simulink library "ProductionLineLib_CM"  (R2025a)
settings: Solver=VariableStepAuto  StartTime=0.0  StopTime=10.0  RelTol=1e-3
libraries: NSA_DEVS_MATH_OPERATIONS x72, $bdroot x37, NSA_DEVS_SOURCES x23, ProductionLineLib_AM x7, NSA_DEVS_DIGITALI3E_CONVERTER x6, NSA_DEVS_STATISTICS x5, NSA_DEVS_QSS x5, NSA_DEVS_ROUTING x4, NSA_DEVS_LOGISTICS x3
(part 1 of 2)
settings Model: Creator=peter  LastModifiedBy=peter
settings RTWCC: GPUComputeCapability=3.5

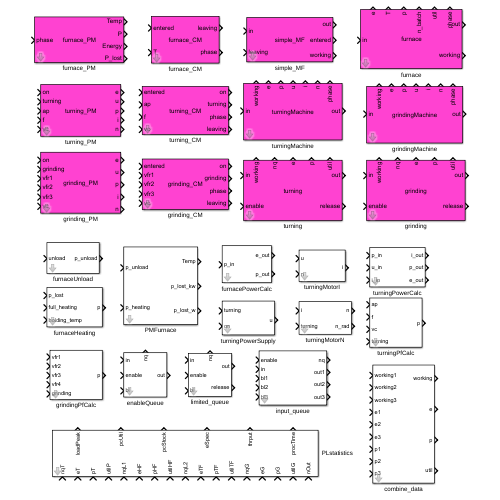
[thumbnail: Simulink's stored preview of the top-level diagram]
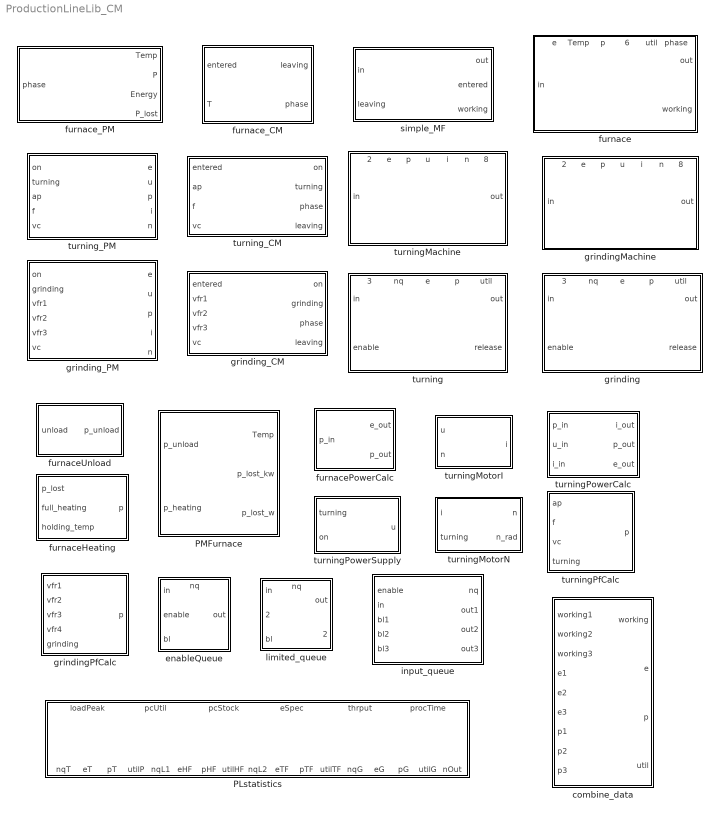
== system ProductionLineLib_CM ==
  PLstatistics : Subsystem  mask{tau=[0,1], debug=0}
      mask DialogControl Container2 Prompt: Advanced
  PMFurnace : Subsystem  mask{Te=0, Co=0, k_A=0, tauInt=[0,100], tau=[0,1], debug=0}
      mask prompts: tauInt "input delay of integrators"
      mask DialogControl Container3 Prompt: General
      mask DialogControl Container2 Prompt: Advanced
  combine_data : Subsystem  mask{tau=[0,1], debug=0}
      mask DialogControl Container3 Prompt: Advanced
  enableQueue : Subsystem  mask{tD=[0,2], tau=[0,1], debug=0}
      mask prompts: tD "delay time of the queuingFree state"
      settings: PortSchema="{\"entries\":[{\"content\":{\"sides\":[{\"content\":{\"connectorIds\":[\"In1\",\"In2\",\"In3\"]},\"type\":\"ConnectorPlacement.EquallySpacedRectSide\",\"uuid\":\"2ad8f87e-7312-4304-b0af-e4f2759959c2\"},{\"content\":{\"connectorIds\":[\"Out1\"],\"side\":\"RIGHT\"},\"type\":\"ConnectorPlacement.EquallySpacedRectSide\",\"uuid\":\"09964865-65de-4b09-b55b-65dbc64d6c80\"},{\"content\":{\"connectorIds\":[\"Out2\"],\"side\":\"TOP\"},\"type\":\"ConnectorPlacement.EquallySpacedRectSide\",\"uuid\":\"570c44b6-46bf-4374-8bed-d6fd4de2ba36\"}]},\"type\":\"ConnectorPlacement.EquallySpacedConnector\",\"uuid\":\"08fead9e-e551-4d6e-a21e-4bd06ec318c1\"}],\"packageUris\":[\"http://schema.mathworks.com/mf0/Connector/R2020b\"],\"version\":\"1.0\"}"
      mask DialogControl Container4 Prompt: Advanced
  furnace : Subsystem  mask{PH=0, Co=0, k_A=0, Te=0, P0=0, P_unload=0, holding_time=0, Tsoll=0, Kapa=0, tauInt=[0,100], tauCont=[0,100], tau=[0,1], debug=0}
      mask prompts: tauInt "input delay of integrators"; tauCont "input delay of controllers"
      settings: PortSchema="{\"entries\":[{\"content\":{\"sides\":[{\"content\":{\"connectorIds\":[\"In1\"]},\"type\":\"ConnectorPlacement.EquallySpacedRectSide\",\"uuid\":\"48eb3c0c-68de-4a57-9b4e-df051f691ee9\"},{\"content\":{\"connectorIds\":[\"Out1\",\"Out2\"],\"side\":\"RIGHT\"},\"type\":\"ConnectorPlacement.EquallySpacedRectSide\",\"uuid\":\"00e094f9-0571-45d6-b681-fd41a6529743\"},{\"content\":{\"connectorIds\":[\"Out3\",\"Out4\",\"Out5\",\"Out6\",\"Out7\",\"Out8\"],\"side\":\"TOP\"},\"type\":\"ConnectorPlacement.EquallySpacedRectSide\",\"uuid\":\"550a95d5-71f4-45dc-b750-a4b185df31ac\"}]},\"type\":\"ConnectorPlacement.EquallySpacedConnector\",\"uuid\":\"8d29a545-a928-42f4-bfc0-37c916a5d15f\"}],\"packageUris\":[\"http://schema.mathworks.com/mf0/Connector/R2020b\"],\"version\":\"1.0\"}"
      mask DialogControl Container2 Prompt: General
      mask DialogControl Container3 Prompt: Advanced
      mask Display:
      | disp('furnace');
      | port_label('input', 1, 'in');
      | 
      | port_label('output', 1, 'out');
      | port_label('output', 2, 'working');
      | port_label('output', 3, 'e');
      | port_label('output', 4, 'T');
      | port_label('output', 5, 'p');
      | port_label('output', 6, 'n_batch');
      | port_label('output', 7, 'util');
      | port_label('output', 8, 'phase');
  furnaceHeating : Subsystem  mask{tau=[0,1], debug=0, PH=0}
      mask DialogControl Container3 Prompt: General
      mask DialogControl Container2 Prompt: Advanced
  furnacePowerCalc : Subsystem  mask{P0=0, tauInt=[0,100], tau=[0,1], debug=0}
      mask prompts: tauInt "input delay of integrators"
      mask DialogControl Container3 Prompt: General
      mask DialogControl Container2 Prompt: Advanced
  furnaceUnload : Subsystem  mask{P_unload=0, tau=[0,1], debug=0}
      mask DialogControl Container3 Prompt: General
      mask DialogControl Container2 Prompt: Advanced
  furnace_CM : Subsystem  mask{holding_time=0, Tsoll=0, tau=[0,1], debug=0}
      mask DialogControl Container2 Prompt: General
      mask DialogControl Container3 Prompt: Advanced
      mask Display:
      | disp('furnace_CM');
      | port_label('input', 1, 'entered');
      | port_label('input', 2, 'T');
      | 
      | port_label('output', 1, 'leaving');
      | port_label('output', 2, 'phase');
  furnace_PM : Subsystem  mask(Furnace_PM){Te=0, P0=0, Co=0, PH=0, k_A=0, P_unload=0, tauInt=[0,100], tauCont=[0,100], tau=[0,1], debug=0}
      mask prompts: tauInt "input delay of integrators"; tauCont "input delay of controllers"
      mask help: Process model of a furnace.
      mask DialogControl Container3 Prompt: General
      mask DialogControl Container2 Prompt: Advanced
      mask Display:
      | disp('furnace_PM');
      | port_label('input', 1, 'phase');
      | 
      | port_label('output', 1, 'Temp');
      | port_label('output', 2, 'P');
      | port_label('output', 3, 'Energy');
      | port_label('output', 4, 'P_lost');
  grinding : Subsystem  mask{vfr1=0.5, vfr2=0.2, vfr3=0.03, vc=10, max_fifo=200, grinding_time=100, tauInt=[0,100], tauCont=[0,100], tau=[0,1], debug=0}
      mask prompts: grinding_time "grinding time"; tauInt "input delay of integrators"; tauCont "input delay of controllers"
      settings: PortSchema="{\"entries\":[{\"content\":{\"sides\":[{\"content\":{\"connectorIds\":[\"In1\",\"In2\"]},\"type\":\"ConnectorPlacement.EquallySpacedRectSide\",\"uuid\":\"33cbe9ec-8ffd-4808-aa33-03a03d7697b3\"},{\"content\":{\"connectorIds\":[\"Out1\",\"Out2\"],\"side\":\"RIGHT\"},\"type\":\"ConnectorPlacement.EquallySpacedRectSide\",\"uuid\":\"c4625700-92c7-457c-b718-8001350e1d76\"},{\"content\":{\"connectorIds\":[\"Out3\",\"Out4\",\"Out5\",\"Out6\",\"Out7\"],\"side\":\"TOP\"},\"type\":\"ConnectorPlacement.EquallySpacedRectSide\",\"uuid\":\"e2440e2f-ad0a-4c1e-a3bb-510435ac270c\"}]},\"type\":\"ConnectorPlacement.EquallySpacedConnector\",\"uuid\":\"8074284e-cd52-45ef-a5c6-c1af8e64b890\"}],\"packageUris\":[\"http://schema.mathworks.com/mf0/Connector/R2020b\"],\"version\":\"1.0\"}"
      mask DialogControl Container2 Prompt: General
      mask DialogControl Container3 Prompt: Advanced
      mask Display:
      | disp('grinding');
      | port_label('input', 1, 'in');
      | port_label('input', 2, 'enable');
      | 
      | port_label('output', 1, 'out');
      | port_label('output', 2, 'release');
      | port_label('output', 3, 'working');
      | port_label('output', 4, 'nq');
      | port_label('output', 5, 'e');
      | port_label('output', 6, 'p');
      | port_label('output', 7, 'util');
  grindingMachine : Subsystem  mask{grinding_time=0, vfr1_ug=0, vfr2_ug=0, vfr3_ug=0, vc_ug=0, vfr1_og=0, vfr2_og=0, vfr3_og=0, vc_og=0, P_vfr1=0, P_vfr2=0, P_vfr3=0, P_vc=0, vfr1=0, vfr2=0, vfr3=0, vc=0, tauInt=[0,100], tauCont=[0,100], tau=[0,1], debug=0}
      mask prompts: tauInt "input delay of integrators"; tauCont "input delay of controllers"
      settings: PortSchema="{\"entries\":[{\"content\":{\"sides\":[{\"content\":{\"connectorIds\":[\"In1\"]},\"type\":\"ConnectorPlacement.EquallySpacedRectSide\",\"uuid\":\"7ed7b3b0-123a-476c-9c35-5e38dde7b955\"},{\"content\":{\"connectorIds\":[\"Out1\"],\"side\":\"RIGHT\"},\"type\":\"ConnectorPlacement.EquallySpacedRectSide\",\"uuid\":\"8397d86f-174e-49cd-8a33-9d60b1d471dc\"},{\"content\":{\"connectorIds\":[\"Out2\",\"Out3\",\"Out4\",\"Out5\",\"Out6\",\"Out7\",\"Out8\"],\"side\":\"TOP\"},\"type\":\"ConnectorPlacement.EquallySpacedRectSide\",\"uuid\":\"d0d4c44f-158b-4425-aa76-17b6d066cd1d\"}]},\"type\":\"ConnectorPlacement.EquallySpacedConnector\",\"uuid\":\"e658c338-98e5-4f30-9f17-73625d396bbf\"}],\"packageUris\":[\"http://schema.mathworks.com/mf0/Connector/R2020b\"],\"version\":\"1.0\"}"
      mask DialogControl Container2 Prompt: General
      mask DialogControl Container3 Prompt: Advanced
      mask Display:
      | disp('grindingMachine');
      | port_label('input', 1, 'in');
      | 
      | port_label('output', 1, 'out');
      | port_label('output', 2, 'working');
      | port_label('output', 3, 'e');
      | port_label('output', 4, 'p');
      | port_label('output', 5, 'u');
      | port_label('output', 6, 'i');
      | port_label('output', 7, 'n');
      | port_label('output', 8, 'phase');
  grindingPfCalc : Subsystem  mask{vfr1_ug=0, vfr1_og=0, P_vfr1=0, vfr2_ug=0, vfr2_og=0, P_vfr2=0, vfr3_ug=0, vfr3_og=0, P_vfr3=0, vc_ug=0, vc_og=0, P_vc=0, tau=[0,1], debug=0}
      mask DialogControl Container3 Prompt: General
      mask DialogControl Container2 Prompt: Advanced
  grinding_CM : Subsystem  mask{grinding_time=0, vfr1_ug=0, vfr2_ug=0, vfr3_ug=0, vc_ug=0, vfr1_og=0, vfr2_og=0, vfr3_og=0, vc_og=0, tau=[0,100], debug=0}
      mask DialogControl Container2 Prompt: General
      mask DialogControl Container3 Prompt: Advanced
      mask Display:
      | disp('grinding_CM');
      | port_label('input', 1, 'entered');
      | port_label('input', 2, 'vfr1');
      | port_label('input', 3, 'vfr2');
      | port_label('input', 4, 'vfr3');
      | port_label('input', 5, 'vc');
      | 
      | port_label('output', 1, 'on');
      | port_label('output', 2, 'grinding');
      | port_label('output', 3, 'phase');
      | port_label('output', 4, 'leaving');
  grinding_PM : Subsystem  mask{R=0, L=0, J=0, b=0, K=0, vcc=0, vcc_load=0, load=0, vfr1_ug=0, vfr2_ug=0, vfr3_ug=0, vc_ug=0, vfr1_og=0, vfr2_og=0, vfr3_og=0, vc_og=0, P_vfr1=0, P_vfr2=0, P_vfr3=0, P_vc=0, tauInt=[0,100], tau=[0,1], debug=0}
      mask prompts: tauInt "input delay of integrators"
      mask DialogControl Container2 Prompt: General
      mask DialogControl Container3 Prompt: Advanced
      mask Display:
      | disp('grinding_PM');
      | port_label('input', 1, 'on');
      | port_label('input', 2, 'grinding');
      | port_label('input', 3, 'vfr1');
      | port_label('input', 4, 'vfr2');
      | port_label('input', 5, 'vfr3');
      | port_label('input', 6, 'vc');
      | 
      | port_label('output', 1, 'e');
      | port_label('output', 2, 'u');
      | port_label('output', 3, 'p');
      | port_label('output', 4, 'i');
      | port_label('output', 5, 'n');
  input_queue : Subsystem  mask{tD=[0,5], tau=[0,5], debug=0}
      mask prompts: tD "delay time of the queuingFree state"
      mask DialogControl Container3 Prompt: Advanced
  limited_queue : Subsystem  mask{max_fifo=400, tD=[0,5], tau=[0,5], debug=0}
      mask prompts: tD "delay time of the queuingFree state"
      settings: PortSchema="{\"entries\":[{\"content\":{\"sides\":[{\"content\":{\"connectorIds\":[\"In1\",\"In2\",\"In3\"]},\"type\":\"ConnectorPlacement.EquallySpacedRectSide\",\"uuid\":\"9e9b3e08-535a-451f-ab10-868cecb889f8\"},{\"content\":{\"connectorIds\":[\"Out1\",\"Out2\"],\"side\":\"RIGHT\"},\"type\":\"ConnectorPlacement.EquallySpacedRectSide\",\"uuid\":\"54afad95-e8b1-4ff2-82f7-3599ee077844\"},{\"content\":{\"connectorIds\":[\"Out3\"],\"side\":\"TOP\"},\"type\":\"ConnectorPlacement.EquallySpacedRectSide\",\"uuid\":\"41a9a62c-ac83-449a-b909-405f9dccd004\"}]},\"type\":\"ConnectorPlacement.EquallySpacedConnector\",\"uuid\":\"98ebd8e6-c994-4b03-9827-f562c62733d8\"}],\"packageUris\":[\"http://schema.mathworks.com/mf0/Connector/R2020b\"],\"version\":\"1.0\"}"
      mask DialogControl Container3 Prompt: General
      mask DialogControl Container2 Prompt: Advanced
  simple_MF : Subsystem  mask{tau=[0,1], debug=0}
      mask DialogControl Container2 Prompt: Advanced
      mask Display:
      | disp('simple_MF');
      | port_label('input', 1, 'in');
      | port_label('input', 2, 'leaving');
      | 
      | port_label('output', 1, 'out');
      | port_label('output', 2, 'entered');
      | port_label('output', 3, 'working');
  turning : Subsystem  mask{ap=1, f=0.1, vc=100, max_fifo=200, turning_time=100, tauInt=[0,100], tauCont=[0,100], tau=[0,1], debug=0}
      mask prompts: turning_time "turning time"; tauInt "input delay of integrators"; tauCont "input delay of controllers"
      settings: PortSchema="{\"entries\":[{\"content\":{\"sides\":[{\"content\":{\"connectorIds\":[\"In1\",\"In2\"]},\"type\":\"ConnectorPlacement.EquallySpacedRectSide\",\"uuid\":\"33cbe9ec-8ffd-4808-aa33-03a03d7697b3\"},{\"content\":{\"connectorIds\":[\"Out1\",\"Out2\"],\"side\":\"RIGHT\"},\"type\":\"ConnectorPlacement.EquallySpacedRectSide\",\"uuid\":\"c4625700-92c7-457c-b718-8001350e1d76\"},{\"content\":{\"connectorIds\":[\"Out3\",\"Out4\",\"Out5\",\"Out6\",\"Out7\"],\"side\":\"TOP\"},\"type\":\"ConnectorPlacement.EquallySpacedRectSide\",\"uuid\":\"e2440e2f-ad0a-4c1e-a3bb-510435ac270c\"}]},\"type\":\"ConnectorPlacement.EquallySpacedConnector\",\"uuid\":\"8074284e-cd52-45ef-a5c6-c1af8e64b890\"}],\"packageUris\":[\"http://schema.mathworks.com/mf0/Connector/R2020b\"],\"version\":\"1.0\"}"
      mask DialogControl Container2 Prompt: General
      mask DialogControl Container3 Prompt: Advanced
      mask Display:
      | disp('turning');
      | port_label('input', 1, 'in');
      | port_label('input', 2, 'enable');
      | 
      | port_label('output', 1, 'out');
      | port_label('output', 2, 'release');
      | port_label('output', 3, 'working');
      | port_label('output', 4, 'nq');
      | port_label('output', 5, 'e');
      | port_label('output', 6, 'p');
      | port_label('output', 7, 'util');
  turningMachine : Subsystem  mask{turning_time=0, ap_ug=0, ap_og=0, P_ap=0, f_ug=0, f_og=0, P_f=0, vc_ug=0, vc_og=0, P_vc=0, ap=0, f=0, vc=0, tauInt=[0,100], tauCont=[0,100], tau=[0,1], debug=0}
      mask prompts: tauInt "input delay of integrators"; tauCont "input delay of controllers"
      settings: PortSchema="{\"entries\":[{\"content\":{\"sides\":[{\"content\":{\"connectorIds\":[\"In1\"]},\"type\":\"ConnectorPlacement.EquallySpacedRectSide\",\"uuid\":\"7ed7b3b0-123a-476c-9c35-5e38dde7b955\"},{\"content\":{\"connectorIds\":[\"Out1\"],\"side\":\"RIGHT\"},\"type\":\"ConnectorPlacement.EquallySpacedRectSide\",\"uuid\":\"8397d86f-174e-49cd-8a33-9d60b1d471dc\"},{\"content\":{\"connectorIds\":[\"Out2\",\"Out3\",\"Out4\",\"Out5\",\"Out6\",\"Out7\",\"Out8\"],\"side\":\"TOP\"},\"type\":\"ConnectorPlacement.EquallySpacedRectSide\",\"uuid\":\"d0d4c44f-158b-4425-aa76-17b6d066cd1d\"}]},\"type\":\"ConnectorPlacement.EquallySpacedConnector\",\"uuid\":\"e658c338-98e5-4f30-9f17-73625d396bbf\"}],\"packageUris\":[\"http://schema.mathworks.com/mf0/Connector/R2020b\"],\"version\":\"1.0\"}"
      mask DialogControl Container2 Prompt: General
      mask DialogControl Container3 Prompt: Advanced
      mask Display:
      | disp('turningMachine');
      | port_label('input', 1, 'in');
      | 
      | port_label('output', 1, 'out');
      | port_label('output', 2, 'working');
      | port_label('output', 3, 'e');
      | port_label('output', 4, 'p');
      | port_label('output', 5, 'u');
      | port_label('output', 6, 'i');
      | port_label('output', 7, 'n');
      | port_label('output', 8, 'phase');
  turningMotorI : Subsystem  mask{R=0, L=0, K=0, tauInt=[0,100], tau=[0,1], debug=0}
      mask prompts: tauInt "input delay of integrators"
      mask DialogControl Container2 Prompt: General
      mask DialogControl Container3 Prompt: Advanced
  turningMotorN : Subsystem  mask{J=0, b=0, K=0, load=0, tauInt=[0,100], tau=[0,1], debug=0}
      mask prompts: tauInt "input delay of integrators"
      mask DialogControl Container2 Prompt: General
      mask DialogControl Container3 Prompt: Advanced
  turningPfCalc : Subsystem  mask{ap_ug=0, ap_og=0, P_ap=0, f_ug=0, f_og=0, P_f=0, vc_ug=0, vc_og=0, P_vc=0, tau=[0,1], debug=0}
      mask DialogControl Container3 Prompt: General
      mask DialogControl Container2 Prompt: Advanced
  turningPowerCalc : Subsystem  mask{tauInt=[0,100], tau=[0,1], debug=0}
      mask prompts: tauInt "input delay of integrators"
      mask DialogControl Container2 Prompt: Advanced
  turningPowerSupply : Subsystem  mask{vcc=0, vcc_load=0, tau=[0,1], debug=0}
      mask DialogControl Container2 Prompt: General
      mask DialogControl Container3 Prompt: Advanced
  turning_CM : Subsystem  mask{turning_time=0, ap_ug=0, f_ug=0, vc_ug=0, ap_og=0, f_og=0, vc_og=0, tau=[0,100], debug=0}
      mask DialogControl Container2 Prompt: General
      mask DialogControl Container3 Prompt: Advanced
      mask Display:
      | disp('turning_CM');
      | port_label('input', 1, 'entered');
      | port_label('input', 2, 'ap');
      | port_label('input', 3, 'f');
      | port_label('input', 4, 'vc');
      | 
      | port_label('output', 1, 'on');
      | port_label('output', 2, 'turning');
      | port_label('output', 3, 'phase');
      | port_label('output', 4, 'leaving');
  turning_PM : Subsystem  mask{R=0, L=0, J=0, b=0, K=0, vcc=0, vcc_load=0, load=0, ap_ug=0, f_ug=0, vc_ug=0, ap_og=0, f_og=0, vc_og=0, P_ap=0, P_f=0, P_vc=0, tauInt=[0,100], tau=[0,1], debug=0}
      mask prompts: tauInt "input delay of integrators"
      mask DialogControl Container2 Prompt: General
      mask DialogControl Container3 Prompt: Advanced
      mask Display:
      | disp('turning_PM');
      | port_label('input', 1, 'on');
      | port_label('input', 2, 'turning');
      | port_label('input', 3, 'ap');
      | port_label('input', 4, 'f');
      | port_label('input', 5, 'vc');
      | 
      | port_label('output', 1, 'e');
      | port_label('output', 2, 'u');
      | port_label('output', 3, 'p');
      | port_label('output', 4, 'i');
      | port_label('output', 5, 'n');

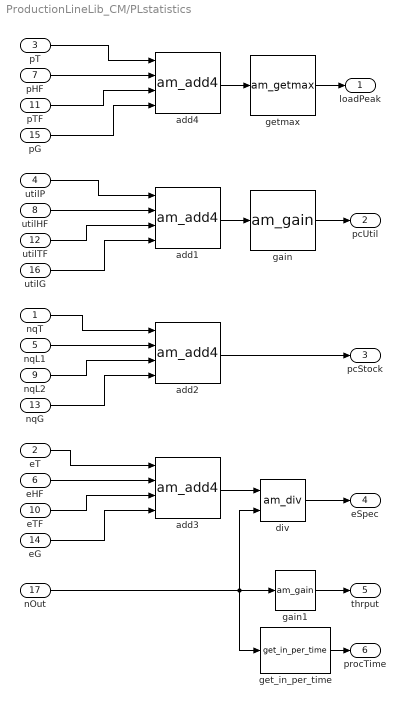
== system ProductionLineLib_CM/PLstatistics ==
  nqT : Inport
  eT : Inport  Port=2
  pT : Inport  Port=3
  utilP : Inport  Port=4
  nqL1 : Inport  Port=5
  eHF : Inport  Port=6
  pHF : Inport  Port=7
  utilHF : Inport  Port=8
  nqL2 : Inport  Port=9
  eTF : Inport  Port=10
  pTF : Inport  Port=11
  utilTF : Inport  Port=12
  nqG : Inport  Port=13
  eG : Inport  Port=14
  pG : Inport  Port=15
  utilG : Inport  Port=16
  nOut : Inport  Port=17
  add{1..4} (4 alike) : NSA_DEVS_MATH_OPERATIONS/am_add4  tau=[0,1]  debug=0
      settings: SourceProductName=Math Operations
  div : NSA_DEVS_MATH_OPERATIONS/am_div  tau=[0,1]  debug=0
      settings: SourceProductName=Math Operations
  gain : NSA_DEVS_MATH_OPERATIONS/am_gain  g=0.25  tau=[0,1]  debug=0
      settings: SourceProductName=Math Operations
  gain1 : NSA_DEVS_MATH_OPERATIONS/am_gain  g=1  tau=[0,1]  debug=0
      settings: SourceProductName=Math Operations
  get_in_per_time : ProductionLineLib_AM/get_in_per_time  tau=[0,1]  debug=0
  getmax : NSA_DEVS_STATISTICS/am_getmax  tau=[0,1]  debug=0
      settings: SourceProductName=Statistics
  loadPeak : Outport
  pcUtil : Outport  Port=2
  pcStock : Outport  Port=3
  eSpec : Outport  Port=4
  thrput : Outport  Port=5
  procTime : Outport  Port=6
  wires:
  pHF/1 -> add4/2
  nqL1/1 -> add2/2
  gain/1 -> pcUtil/1
  utilHF/1 -> add1/2
  add4/1 -> getmax/1
  eG/1 -> add3/4
  nOut/1 -> gain1/1, get_in_per_time/1, div/2
  utilTF/1 -> add1/3
  utilP/1 -> add1/1
  eHF/1 -> add3/2
  eT/1 -> add3/1
  add2/1 -> pcStock/1
  add1/1 -> gain/1
  pTF/1 -> add4/3
  nqT/1 -> add2/1
  nqL2/1 -> add2/3
  eTF/1 -> add3/3
  pG/1 -> add4/4
  pT/1 -> add4/1
  nqG/1 -> add2/4
  utilG/1 -> add1/4
  div/1 -> eSpec/1
  getmax/1 -> loadPeak/1
  add3/1 -> div/1
  get_in_per_time/1 -> procTime/1
  gain1/1 -> thrput/1

== system ProductionLineLib_CM/PMFurnace ==
  p_unload : Inport
  p_heating : Inport  Port=2
  add3 : NSA_DEVS_MATH_OPERATIONS/am_add3  tau=tau  debug=debug
      settings: SourceProductName=Math Operations
  am_add2 : NSA_DEVS_MATH_OPERATIONS/am_add2  tau=[0,1]  debug=0
      settings: SourceProductName=Math Operations
  am_const : NSA_DEVS_SOURCES/am_const  value=-Te  sendTime=[0,1]  debug=0
      settings: SourceProductName=Sources
  gain : NSA_DEVS_MATH_OPERATIONS/am_gain  g=1/Co  tau=[0,1]  debug=debug
      settings: SourceProductName=Math Operations
  gain1 : NSA_DEVS_MATH_OPERATIONS/am_gain  g=k_A  tau=[0,1]  debug=debug
      settings: SourceProductName=Math Operations
  gain2 : NSA_DEVS_MATH_OPERATIONS/am_gain  g=1/1000  tau=[0,1]  debug=debug
      settings: SourceProductName=Math Operations
  gain3 : NSA_DEVS_MATH_OPERATIONS/am_gain  g=-1  tau=[0,1]  debug=debug
      settings: SourceProductName=Math Operations
  hIntegrator : NSA_DEVS_QSS/am_hIntegrator  dq=25  epsilon=25  X0=Te  tau=tauInt  debug=debug
      settings: SourceProductName=QSS
  Temp : Outport
  p_lost_kw : Outport  Port=2
  p_lost_w : Outport  Port=3
  wires:
  hIntegrator/1 -> am_add2/2, Temp/1
  p_heating/1 -> add3/2
  p_unload/1 -> add3/1
  gain3/1 -> add3/3
  gain2/1 -> p_lost_kw/1
  am_add2/1 -> gain1/1
  gain1/1 -> gain2/1, p_lost_w/1, gain3/1
  am_const/1 -> am_add2/1
  gain/1 -> hIntegrator/1
  add3/1 -> gain/1

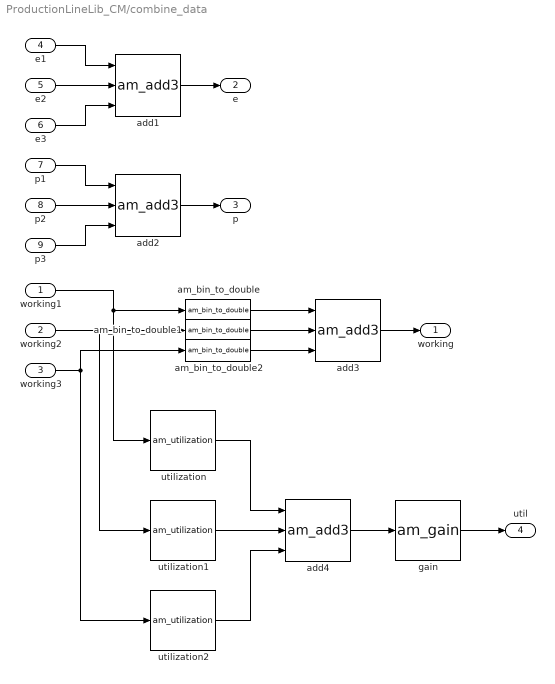
== system ProductionLineLib_CM/combine_data ==
  working1 : Inport
  working2 : Inport  Port=2
  working3 : Inport  Port=3
  e1 : Inport  Port=4
  e2 : Inport  Port=5
  e3 : Inport  Port=6
  p1 : Inport  Port=7
  p2 : Inport  Port=8
  p3 : Inport  Port=9
  add{1..4} (4 alike) : NSA_DEVS_MATH_OPERATIONS/am_add3  tau=[0,1]  debug=0
      settings: SourceProductName=Math Operations
  am_bin_to_double : NSA_DEVS_DIGITALI3E_CONVERTER/am_bin_to_double  tau=[0,1]  debug=0
  am_bin_to_double1 : NSA_DEVS_DIGITALI3E_CONVERTER/am_bin_to_double  tau=[0,1]  debug=0
  am_bin_to_double2 : NSA_DEVS_DIGITALI3E_CONVERTER/am_bin_to_double  tau=[0,1]  debug=0
  gain : NSA_DEVS_MATH_OPERATIONS/am_gain  g=1/3  tau=[0,1]  debug=0
      settings: SourceProductName=Math Operations
  utilization : NSA_DEVS_STATISTICS/am_utilization  tau=[0,1]  debug=0
      settings: SourceProductName=Statistics
  utilization1 : NSA_DEVS_STATISTICS/am_utilization  tau=[0,1]  debug=0
      settings: SourceProductName=Statistics
  utilization2 : NSA_DEVS_STATISTICS/am_utilization  tau=[0,1]  debug=0
      settings: SourceProductName=Statistics
  working : Outport
  e : Outport  Port=2
  p : Outport  Port=3
  util : Outport  Port=4
  wires:
  working2/1 -> utilization1/1, am_bin_to_double1/1
  working1/1 -> am_bin_to_double/1, utilization/1
  working3/1 -> am_bin_to_double2/1, utilization2/1
  add3/1 -> working/1
  e2/1 -> add1/2
  add1/1 -> e/1
  e1/1 -> add1/1
  e3/1 -> add1/3
  p2/1 -> add2/2
  p1/1 -> add2/1
  p3/1 -> add2/3
  add2/1 -> p/1
  utilization1/1 -> add4/2
  utilization/1 -> add4/1
  utilization2/1 -> add4/3
  add4/1 -> gain/1
  gain/1 -> util/1
  am_bin_to_double/1 -> add3/1
  am_bin_to_double1/1 -> add3/2
  am_bin_to_double2/1 -> add3/3

== system ProductionLineLib_CM/enableQueue ==
  in : Inport
  enable : Inport  Port=2
  bl : Inport  Port=3
  am_not1 : NSA_DEVS_MATH_OPERATIONS/am_not  i0=true  tau_copy=[0,1]  debug_copy=0
      settings: SourceProductName=Math Operations
  am_or2 : NSA_DEVS_MATH_OPERATIONS/am_or2  i0=false  tau_copy=[0,1]  debug_copy=0
      settings: SourceProductName=Math Operations
  queue : NSA_DEVS_LOGISTICS/am_queue  tD=tD  tau=tau  debug=debug
      settings: SourceProductName=Logistics
  out : Outport
  nq : Outport  Port=2
  wires:
  enable/1 -> am_not1/1
  am_not1/1 -> am_or2/1
  bl/1 -> am_or2/2
  in/1 -> queue/1
  am_or2/1 -> queue/2
  queue/1 -> out/1
  queue/2 -> nq/1

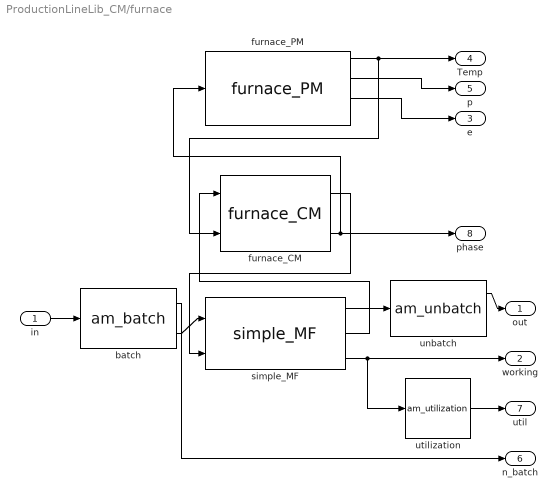
== system ProductionLineLib_CM/furnace ==
  in : Inport
  batch : NSA_DEVS_LOGISTICS/am_batch  N=Kapa  tau=tau  debug=debug
      settings: SourceProductName=Logistics
  furnace_CM : $bdroot/furnace_CM  holding_time=holding_time  Tsoll=Tsoll  tau=tauCont  debug=debug
  furnace_PM : $bdroot/furnace_PM  Te=Te  P0=P0  Co=Co  PH=PH  k_A=k_A  P_unload=P_unload  tauInt=tauInt  tauCont=tauCont  tau=[0,1]  debug=debug
  simple_MF : $bdroot/simple_MF  tau=[0,1]  debug=debug
      settings: LibrarySourceBlock=ProductionLineLib_CM/furnace_MF
  unbatch : NSA_DEVS_LOGISTICS/am_unbatch  tD=[0,100]  tau=[0,100]  debug=debug
      settings: SourceProductName=Logistics
  utilization : NSA_DEVS_STATISTICS/am_utilization  tau=[0,1]  debug=debug
      settings: SourceProductName=Statistics
  out : Outport
  working : Outport  Port=2
  e : Outport  Port=3
  Temp : Outport  Port=4
  p : Outport  Port=5
  n_batch : Outport  Port=6
  util : Outport  Port=7
  phase : Outport  Port=8
  wires:
  furnace_CM/1 -> simple_MF/2
  simple_MF/2 -> furnace_CM/1
  furnace_CM/2 -> phase/1, furnace_PM/1
  furnace_PM/2 -> p/1
  furnace_PM/3 -> e/1
  furnace_PM/1 -> Temp/1, furnace_CM/2
  batch/2 -> n_batch/1
  utilization/1 -> util/1
  simple_MF/3 -> utilization/1, working/1
  unbatch/1 -> out/1
  simple_MF/1 -> unbatch/1
  batch/1 -> simple_MF/1
  in/1 -> batch/1

== system ProductionLineLib_CM/furnaceHeating ==
  p_lost : Inport
  full_heating : Inport  Port=2
  holding_temp : Inport  Port=3
  am_add2 : NSA_DEVS_MATH_OPERATIONS/am_add2  tau=[0,1]  debug=0
      settings: SourceProductName=Math Operations
  am_gain : NSA_DEVS_MATH_OPERATIONS/am_gain  g=PH  tau=[0,1]  debug=0
      settings: SourceProductName=Math Operations
  am_multi2 : NSA_DEVS_MATH_OPERATIONS/am_mult2  tau=[0,1]  debug=0
      settings: SourceProductName=Math Operations
  p : Outport
  wires:
  full_heating/1 -> am_gain/1
  am_gain/1 -> am_add2/2
  p_lost/1 -> am_multi2/2
  am_add2/1 -> p/1
  holding_temp/1 -> am_multi2/1
  am_multi2/1 -> am_add2/1

== system ProductionLineLib_CM/furnacePowerCalc ==
  p_in : Inport
  add2 : NSA_DEVS_MATH_OPERATIONS/am_add2  tau=tau  debug=debug
      settings: SourceProductName=Math Operations
  const : NSA_DEVS_SOURCES/am_const  value=P0  sendTime=[0,1]  debug=debug
      settings: SourceProductName=Sources
  gain : NSA_DEVS_MATH_OPERATIONS/am_gain  g=1/3600  tau=[0,1]  debug=debug
      settings: SourceProductName=Math Operations
  gain1 : NSA_DEVS_MATH_OPERATIONS/am_gain  g=1/1000  tau=[0,1]  debug=debug
      settings: SourceProductName=Math Operations
  hIntegrator : NSA_DEVS_QSS/am_hIntegrator  dq=0.1  epsilon=0.1  X0=0  tau=tauInt  debug=debug
      settings: SourceProductName=QSS
  e_out : Outport
  p_out : Outport  Port=2
  wires:
  p_in/1 -> add2/1
  gain/1 -> hIntegrator/1
  hIntegrator/1 -> e_out/1
  gain1/1 -> p_out/1, gain/1
  add2/1 -> gain1/1
  const/1 -> add2/2

== system ProductionLineLib_CM/furnaceUnload ==
  unload : Inport
  am_const : NSA_DEVS_SOURCES/am_const  value=P_unload  sendTime=[0,1]  debug=0
      settings: SourceProductName=Sources
  am_gain : NSA_DEVS_MATH_OPERATIONS/am_gain  g=-1  tau=[0,1]  debug=0
      settings: SourceProductName=Math Operations
  am_multi2 : NSA_DEVS_MATH_OPERATIONS/am_mult2  tau=[0,1]  debug=0
      settings: SourceProductName=Math Operations
  p_unload : Outport
  wires:
  am_const/1 -> am_multi2/2
  am_gain/1 -> p_unload/1
  unload/1 -> am_multi2/1
  am_multi2/1 -> am_gain/1

== system ProductionLineLib_CM/furnace_CM ==
  entered : Inport
  T : Inport  Port=2
  checkTemperature1 : ProductionLineLib_AM/checkTemperature  tau=tau  debug=debug
  furnace_controller : ProductionLineLib_AM/furnace_controller  holding_time=holding_time  Tsoll=Tsoll  tau=tau  debug=debug
      settings: LibrarySourceBlock=ProductionLineLib/Atomics/furnacs_controller
  leaving : Outport
  phase : Outport  Port=2
  wires:
  furnace_controller/3 -> checkTemperature1/3
  checkTemperature1/1 -> furnace_controller/2
  furnace_controller/2 -> checkTemperature1/1, phase/1
  furnace_controller/1 -> leaving/1
  T/1 -> checkTemperature1/2
  entered/1 -> furnace_controller/1

== system ProductionLineLib_CM/furnace_PM ==
  phase : Inport
  PMFurnace : $bdroot/PMFurnace  Te=Te  Co=Co  k_A=k_A  tauInt=tauInt  tau=[0,1]  debug=debug
      settings: LibrarySourceBlock=ProductionLineLib_CM/PM_furnace
  furnaceHeating : $bdroot/furnaceHeating  tau=[0,1]  debug=debug  PH=PH
      settings: LibrarySourceBlock=ProductionLineLib_CM/PM_heating
  furnacePowerCalc : $bdroot/furnacePowerCalc  P0=P0  tauInt=tauInt  tau=[0,1]  debug=debug
      settings: LibrarySourceBlock=ProductionLineLib_CM/PM_power_calc
  furnaceUnload : $bdroot/furnaceUnload  P_unload=P_unload  tau=[0,1]  debug=debug
  heat_controller : ProductionLineLib_AM/heat_controller  tau=tauCont  debug=debug
      settings: LibrarySourceBlock=ProductionLineLibAM/heatController
  Temp : Outport
  P : Outport  Port=2
  Energy : Outport  Port=3
  P_lost : Outport  Port=4
  wires:
  furnaceUnload/1 -> PMFurnace/1
  heat_controller/3 -> furnaceUnload/1
  PMFurnace/2 -> P_lost/1
  PMFurnace/3 -> furnaceHeating/1
  PMFurnace/1 -> Temp/1
  heat_controller/2 -> furnaceHeating/3
  heat_controller/1 -> furnaceHeating/2
  furnaceHeating/1 -> PMFurnace/2, furnacePowerCalc/1
  furnacePowerCalc/2 -> P/1
  furnacePowerCalc/1 -> Energy/1
  phase/1 -> heat_controller/1

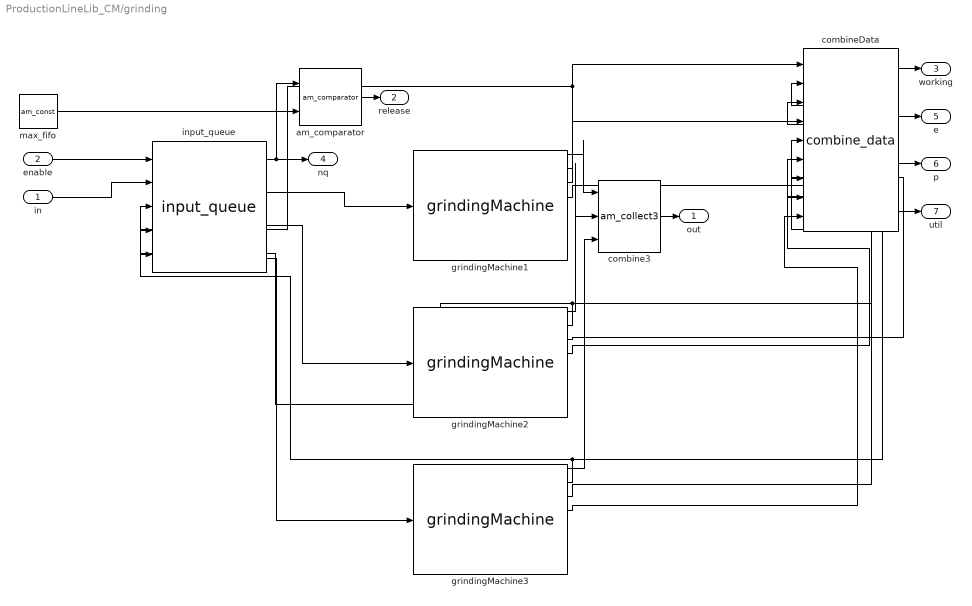
== system ProductionLineLib_CM/grinding ==
  in : Inport
  enable : Inport  Port=2
  am_comparator : NSA_DEVS_MATH_OPERATIONS/am_comparator  compop="\"<\""  tau=[0,1]  debug=0
      settings: SourceProductName=Math Operations
  combine3 : NSA_DEVS_ROUTING/am_collect3  tD=[0,10]  tau=[0,1]  debug=debug
      settings: SourceProductName=Routing
  combineData : $bdroot/combine_data  tau=[0,1]  debug=0
  grindingMachine1 : $bdroot/grindingMachine  grinding_time=grinding_time  vfr1_ug=0.48  vfr2_ug=0.19  vfr3_ug=0.03  vc_ug=30  vfr1_og=1.86  vfr2_og=0.53  vfr3_og=0.16  vc_og=50  P_vfr1=0.2  P_vfr2=0.2  P_vfr3=0.2  P_vc=0.6  vfr1=vfr1  vfr2=vfr2  vfr3=vfr3  vc=vc  tauInt=tauInt  tauCont=tauCont  tau=[0,1]  debug=0
  grindingMachine2 : $bdroot/grindingMachine  grinding_time=grinding_time  vfr1_ug=0.48  vfr2_ug=0.19  vfr3_ug=0.03  vc_ug=30  vfr1_og=1.86  vfr2_og=0.53  vfr3_og=0.16  vc_og=50  P_vfr1=0.2  P_vfr2=0.2  P_vfr3=0.2  P_vc=0.6  vfr1=vfr1  vfr2=vfr2  vfr3=vfr3  vc=vc  tauInt=tauInt  tauCont=tauCont  tau=[0,1]  debug=0
  grindingMachine3 : $bdroot/grindingMachine  grinding_time=grinding_time  vfr1_ug=0.48  vfr2_ug=0.19  vfr3_ug=0.03  vc_ug=30  vfr1_og=1.86  vfr2_og=0.53  vfr3_og=0.16  vc_og=50  P_vfr1=0.2  P_vfr2=0.2  P_vfr3=0.2  P_vc=0.6  vfr1=vfr1  vfr2=vfr2  vfr3=vfr3  vc=vc  tauInt=tauInt  tauCont=tauCont  tau=[0,1]  debug=0
  input_queue : $bdroot/input_queue  tD=[0,5]  tau=[0,5]  debug=debug
  max_fifo : NSA_DEVS_SOURCES/am_const  value=max_fifo  sendTime=[0,1]  debug=debug
      settings: SourceProductName=Sources
  out : Outport
  release : Outport  Port=2
  working : Outport  Port=3
  nq : Outport  Port=4
  e : Outport  Port=5
  p : Outport  Port=6
  util : Outport  Port=7
  wires:
  grindingMachine2/2 -> input_queue/4, combineData/2
  grindingMachine1/2 -> input_queue/3, combineData/1
  grindingMachine1/1 -> combine3/1
  grindingMachine2/1 -> combine3/2
  grindingMachine3/1 -> combine3/3
  combine3/1 -> out/1
  grindingMachine3/2 -> input_queue/5, combineData/3
  enable/1 -> input_queue/1
  in/1 -> input_queue/2
  input_queue/1 -> am_comparator/1, nq/1
  input_queue/2 -> grindingMachine1/1
  input_queue/3 -> grindingMachine2/1
  input_queue/4 -> grindingMachine3/1
  grindingMachine1/3 -> combineData/4
  grindingMachine1/4 -> combineData/7
  grindingMachine2/3 -> combineData/5
  grindingMachine2/4 -> combineData/8
  grindingMachine3/3 -> combineData/6
  grindingMachine3/4 -> combineData/9
  combineData/1 -> working/1
  combineData/3 -> p/1
  combineData/2 -> e/1
  combineData/4 -> util/1
  am_comparator/1 -> release/1
  max_fifo/1 -> am_comparator/2

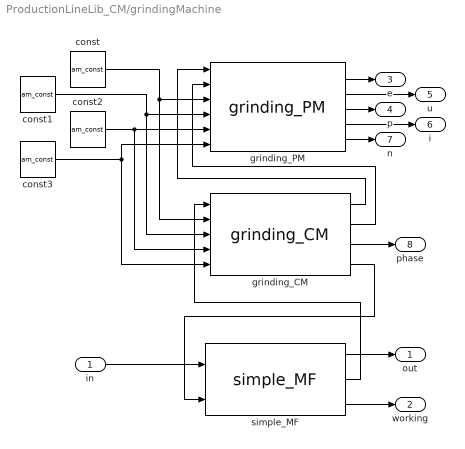
== system ProductionLineLib_CM/grindingMachine ==
  in : Inport
  const : NSA_DEVS_SOURCES/am_const  value=vfr1  sendTime=[0,1]  debug=0
      settings: SourceProductName=Sources
  const1 : NSA_DEVS_SOURCES/am_const  value=vfr2  sendTime=[0,1]  debug=0
      settings: SourceProductName=Sources
  const2 : NSA_DEVS_SOURCES/am_const  value=vfr3  sendTime=[0,1]  debug=0
      settings: SourceProductName=Sources
  const3 : NSA_DEVS_SOURCES/am_const  value=vc  sendTime=[0,1]  debug=0
      settings: SourceProductName=Sources
  grinding_CM : $bdroot/grinding_CM  grinding_time=grinding_time  vfr1_ug=vfr1_ug  vfr2_ug=vfr2_ug  vfr3_ug=vfr3_ug  vc_ug=vc_ug  vfr1_og=vfr1_og  vfr2_og=vfr2_og  vfr3_og=vfr3_og  vc_og=vc_og  tau=tauCont  debug=debug
  grinding_PM : $bdroot/grinding_PM  R=6  L=0.2  J=0.052  b=0.015  K=0.15  vcc=150  vcc_load=30  load=0.75/200  vfr1_ug=vfr1_ug  vfr2_ug=vfr2_ug  vfr3_ug=vfr3_ug  vc_ug=vc_ug  vfr1_og=vfr1_og  vfr2_og=vfr2_og  vfr3_og=vfr3_og  vc_og=vc_og  P_vfr1=P_vfr1  P_vfr2=P_vfr2  P_vfr3=P_vfr3  P_vc=P_vc  tauInt=tauInt  tau=tau  debug=debug
  simple_MF : $bdroot/simple_MF  tau=tau  debug=debug
  out : Outport
  working : Outport  Port=2
  e : Outport  Port=3
  p : Outport  Port=4
  u : Outport  Port=5
  i : Outport  Port=6
  n : Outport  Port=7
  phase : Outport  Port=8
  wires:
  grinding_CM/3 -> phase/1
  grinding_PM/5 -> n/1
  grinding_PM/4 -> i/1
  grinding_PM/2 -> u/1
  in/1 -> simple_MF/1
  simple_MF/1 -> out/1
  simple_MF/3 -> working/1
  grinding_PM/1 -> e/1
  grinding_PM/3 -> p/1
  grinding_CM/1 -> grinding_PM/1
  grinding_CM/2 -> grinding_PM/2
  grinding_CM/4 -> simple_MF/2
  simple_MF/2 -> grinding_CM/1
  const/1 -> grinding_CM/2, grinding_PM/3
  const1/1 -> grinding_CM/3, grinding_PM/4
  const3/1 -> grinding_PM/6, grinding_CM/5
  const2/1 -> grinding_CM/4, grinding_PM/5

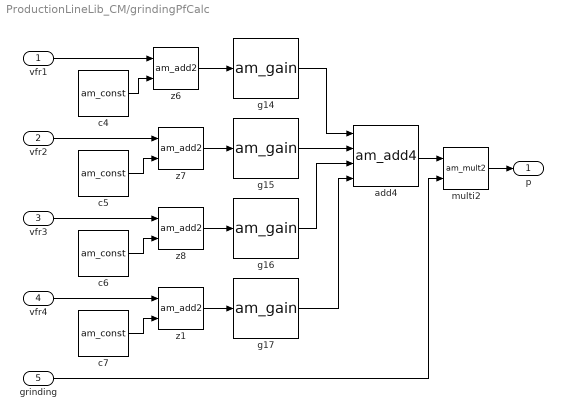
== system ProductionLineLib_CM/grindingPfCalc ==
  vfr1 : Inport
  vfr2 : Inport  Port=2
  vfr3 : Inport  Port=3
  vfr4 : Inport  Port=4
  grinding : Inport  Port=5
  add4 : NSA_DEVS_MATH_OPERATIONS/am_add4  tau=[0,1]  debug=debug
      settings: SourceProductName=Math Operations
  c4 : NSA_DEVS_SOURCES/am_const  value=vfr1_ug  sendTime=[0,1]  debug=debug
      settings: SourceProductName=Sources
  c5 : NSA_DEVS_SOURCES/am_const  value=vfr2_ug  sendTime=[0,1]  debug=debug
      settings: SourceProductName=Sources
  c6 : NSA_DEVS_SOURCES/am_const  value=vfr3_ug  sendTime=[0,1]  debug=debug
      settings: SourceProductName=Sources
  c7 : NSA_DEVS_SOURCES/am_const  value=vc_ug  sendTime=[0,1]  debug=debug
      settings: SourceProductName=Sources
  g14 : NSA_DEVS_MATH_OPERATIONS/am_gain  g=1/(vfr1_og-vfr1_ug)*P_vfr1  tau=[0,1]  debug=debug
      settings: SourceProductName=Math Operations
  g15 : NSA_DEVS_MATH_OPERATIONS/am_gain  g=1/(vfr2_og-vfr2_ug)*P_vfr2  tau=[0,1]  debug=debug
      settings: SourceProductName=Math Operations
  g16 : NSA_DEVS_MATH_OPERATIONS/am_gain  g=1/(vfr3_og-vfr3_ug)*P_vfr3  tau=[0,1]  debug=debug
      settings: SourceProductName=Math Operations
  g17 : NSA_DEVS_MATH_OPERATIONS/am_gain  g=1/(vc_og-vc_ug)*P_vc  tau=[0,1]  debug=debug
      settings: SourceProductName=Math Operations
  multi2 : NSA_DEVS_MATH_OPERATIONS/am_mult2  tau=tau  debug=debug
      settings: SourceProductName=Math Operations
  z{1,6..8} (4 alike) : NSA_DEVS_MATH_OPERATIONS/am_add2  tau=tau  debug=debug
      settings: SourceProductName=Math Operations
  p : Outport
  wires:
  vfr2/1 -> z7/1
  vfr1/1 -> z6/1
  add4/1 -> multi2/1
  vfr3/1 -> z8/1
  c5/1 -> z7/2
  multi2/1 -> p/1
  z7/1 -> g15/1
  c4/1 -> z6/2
  z6/1 -> g14/1
  grinding/1 -> multi2/2
  g16/1 -> add4/3
  z8/1 -> g16/1
  c6/1 -> z8/2
  g15/1 -> add4/2
  g14/1 -> add4/1
  c7/1 -> z1/2
  z1/1 -> g17/1
  g17/1 -> add4/4
  vfr4/1 -> z1/1

== system ProductionLineLib_CM/grinding_CM ==
  entered : Inport
  vfr1 : Inport  Port=2
  vfr2 : Inport  Port=3
  vfr3 : Inport  Port=4
  vc : Inport  Port=5
  grinding_controller : ProductionLineLib_AM/grinding_controller  grinding_time=grinding_time  vfr1_ug=vfr1_ug  vfr2_ug=vfr2_ug  vfr3_ug=vfr3_ug  vc_ug=vc_ug  vfr1_og=vfr1_og  vfr2_og=vfr2_og  vfr3_og=vfr3_og  vc_og=vc_og  tau=tau  debug=debug
  on : Outport
  grinding : Outport  Port=2
  phase : Outport  Port=3
  leaving : Outport  Port=4
  wires:
  vc/1 -> grinding_controller/5
  vfr3/1 -> grinding_controller/4
  vfr2/1 -> grinding_controller/3
  vfr1/1 -> grinding_controller/2
  grinding_controller/3 -> phase/1
  grinding_controller/2 -> grinding/1
  grinding_controller/1 -> on/1
  entered/1 -> grinding_controller/1
  grinding_controller/4 -> leaving/1

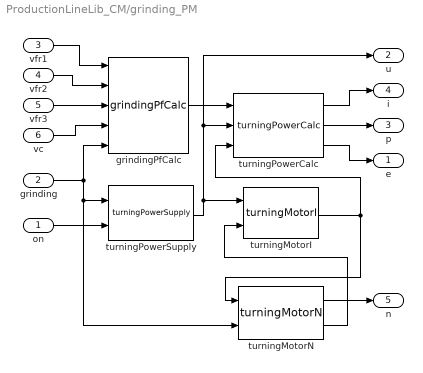
== system ProductionLineLib_CM/grinding_PM ==
  on : Inport
  grinding : Inport  Port=2
  vfr1 : Inport  Port=3
  vfr2 : Inport  Port=4
  vfr3 : Inport  Port=5
  vc : Inport  Port=6
  grindingPfCalc : $bdroot/grindingPfCalc  vfr1_ug=vfr1_ug  vfr1_og=vfr1_og  P_vfr1=P_vfr1  vfr2_ug=vfr2_ug  vfr2_og=vfr2_og  P_vfr2=P_vfr2  vfr3_ug=vfr3_ug  vfr3_og=vfr3_og  P_vfr3=P_vfr3  vc_ug=vc_ug  vc_og=vc_og  P_vc=P_vc  tau=tau  debug=debug
  turningMotorI : $bdroot/turningMotorI  R=R  L=L  K=K  tauInt=tauInt  tau=[0,1]  debug=debug
  turningMotorN : $bdroot/turningMotorN  J=J  b=b  K=K  load=load  tauInt=tauInt  tau=[0,1]  debug=debug
  turningPowerCalc : $bdroot/turningPowerCalc  tauInt=tauInt  tau=[0,1]  debug=debug
  turningPowerSupply : $bdroot/turningPowerSupply  vcc=vcc  vcc_load=vcc_load  tau=tau  debug=debug
  e : Outport
  u : Outport  Port=2
  p : Outport  Port=3
  i : Outport  Port=4
  n : Outport  Port=5
  wires:
  on/1 -> turningPowerSupply/2
  turningPowerSupply/1 -> turningPowerCalc/2, u/1, turningMotorI/1
  turningMotorN/2 -> turningMotorI/2
  turningMotorN/1 -> n/1
  turningMotorI/1 -> turningPowerCalc/3, turningMotorN/1
  turningPowerCalc/3 -> e/1
  turningPowerCalc/2 -> p/1
  turningPowerCalc/1 -> i/1
  grindingPfCalc/1 -> turningPowerCalc/1
  vc/1 -> grindingPfCalc/4
  vfr3/1 -> grindingPfCalc/3
  vfr2/1 -> grindingPfCalc/2
  vfr1/1 -> grindingPfCalc/1
  grinding/1 -> turningMotorN/2, turningPowerSupply/1, grindingPfCalc/5

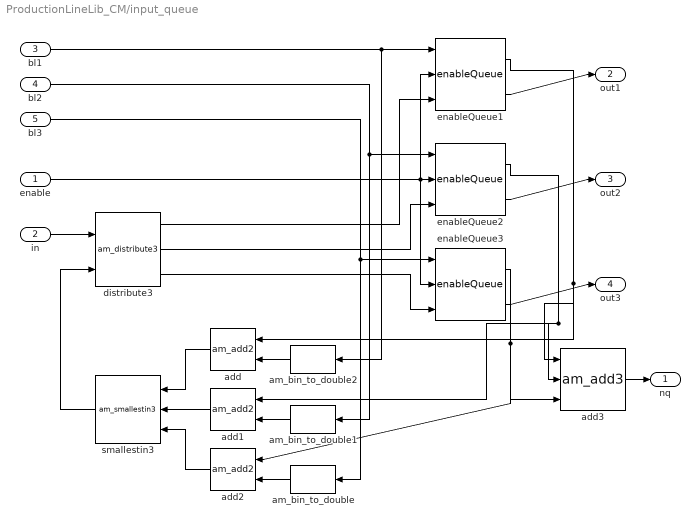
== system ProductionLineLib_CM/input_queue ==
  enable : Inport
  in : Inport  Port=2
  bl1 : Inport  Port=3
  bl2 : Inport  Port=4
  bl3 : Inport  Port=5
  add : NSA_DEVS_MATH_OPERATIONS/am_add2  tau=[0,1]  debug=debug
      settings: SourceProductName=Math Operations
  add1 : NSA_DEVS_MATH_OPERATIONS/am_add2  tau=[0,1]  debug=debug
      settings: SourceProductName=Math Operations
  add2 : NSA_DEVS_MATH_OPERATIONS/am_add2  tau=[0,1]  debug=debug
      settings: SourceProductName=Math Operations
  add3 : NSA_DEVS_MATH_OPERATIONS/am_add3  tau=[0,1]  debug=debug
      settings: SourceProductName=Math Operations
  am_bin_to_double : NSA_DEVS_DIGITALI3E_CONVERTER/am_bin_to_double  tau=[0,1]  debug=0
  am_bin_to_double1 : NSA_DEVS_DIGITALI3E_CONVERTER/am_bin_to_double  tau=[0,1]  debug=0
  am_bin_to_double2 : NSA_DEVS_DIGITALI3E_CONVERTER/am_bin_to_double  tau=[0,1]  debug=0
  distribute3 : NSA_DEVS_ROUTING/am_distribute3  port0=1  field="\"\""  tau=[0,10]  debug=debug
      settings: SourceProductName=Routing
  enableQueue1 : $bdroot/enableQueue  tD=tD  tau=tau  debug=debug
  enableQueue2 : $bdroot/enableQueue  tD=tD  tau=tau  debug=debug
  enableQueue3 : $bdroot/enableQueue  tD=tD  tau=tau  debug=debug
  smallestin3 : NSA_DEVS_ROUTING/am_smallestin3  val0=0  tau=[0,1]  debug=debug
      settings: SourceProductName=Routing
  nq : Outport
  out1 : Outport  Port=2
  out2 : Outport  Port=3
  out3 : Outport  Port=4
  wires:
  bl1/1 -> am_bin_to_double2/1, enableQueue1/3
  bl2/1 -> enableQueue2/3, am_bin_to_double1/1
  bl3/1 -> am_bin_to_double/1, enableQueue3/3
  enable/1 -> enableQueue3/2, enableQueue1/2, enableQueue2/2
  in/1 -> distribute3/1
  distribute3/3 -> enableQueue3/1
  distribute3/2 -> enableQueue2/1
  distribute3/1 -> enableQueue1/1
  smallestin3/1 -> distribute3/2
  enableQueue3/2 -> add3/3, add2/1
  enableQueue2/2 -> add1/1, add3/2
  enableQueue1/2 -> add3/1, add/1
  enableQueue1/1 -> out1/1
  enableQueue2/1 -> out2/1
  enableQueue3/1 -> out3/1
  add3/1 -> nq/1
  add1/1 -> smallestin3/2
  add/1 -> smallestin3/1
  add2/1 -> smallestin3/3
  am_bin_to_double/1 -> add2/2
  am_bin_to_double1/1 -> add1/2
  am_bin_to_double2/1 -> add/2

== system ProductionLineLib_CM/limited_queue ==
  in : Inport
  enable : Inport  Port=2
  bl : Inport  Port=3
  am_comparator : NSA_DEVS_MATH_OPERATIONS/am_comparator  compop="\"<\""  tau=[0,1]  debug=0
      settings: SourceProductName=Math Operations
  enableQueue : $bdroot/enableQueue  tD=tD  tau=tau  debug=debug
  max_fifo : NSA_DEVS_SOURCES/am_const  value=max_fifo  sendTime=[0,1]  debug=0
      settings: SourceProductName=Sources
  out : Outport
  release : Outport  Port=2
  nq : Outport  Port=3
  wires:
  in/1 -> enableQueue/1
  enable/1 -> enableQueue/2
  bl/1 -> enableQueue/3
  enableQueue/1 -> out/1
  enableQueue/2 -> am_comparator/1, nq/1
  max_fifo/1 -> am_comparator/2
  am_comparator/1 -> release/1

== system ProductionLineLib_CM/simple_MF ==
  in : Inport
  leaving : Inport  Port=2
  triggeredserver : ProductionLineLib_AM/triggeredserver  tau=tau  debug=debug
      settings: LibrarySourceBlock=ProductionLineLib_AM/furnace_server
  out : Outport
  entered : Outport  Port=2
  working : Outport  Port=3
  wires:
  in/1 -> triggeredserver/1
  leaving/1 -> triggeredserver/2
  triggeredserver/1 -> out/1
  triggeredserver/2 -> entered/1
  triggeredserver/3 -> working/1

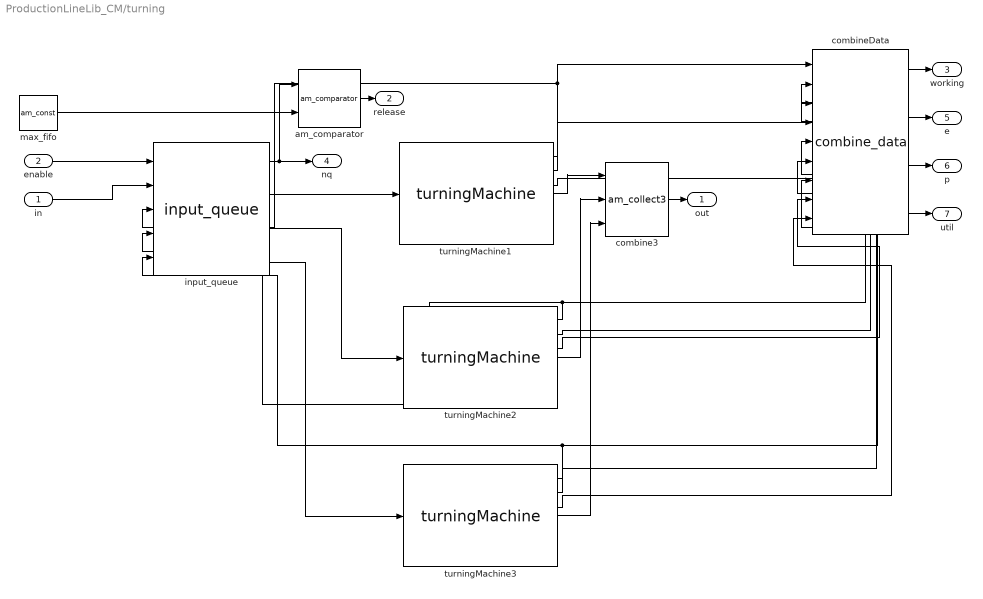
== system ProductionLineLib_CM/turning ==
  in : Inport
  enable : Inport  Port=2
  am_comparator : NSA_DEVS_MATH_OPERATIONS/am_comparator  compop="\"<\""  tau=[0,1]  debug=0
      settings: SourceProductName=Math Operations
  combine3 : NSA_DEVS_ROUTING/am_collect3  tD=[0,10]  tau=[0,1]  debug=debug
      settings: SourceProductName=Routing
  combineData : $bdroot/combine_data  tau=[0,1]  debug=0
  input_queue : $bdroot/input_queue  tD=[0,5]  tau=[0,5]  debug=debug
  max_fifo : NSA_DEVS_SOURCES/am_const  value=max_fifo  sendTime=[0,1]  debug=debug
      settings: SourceProductName=Sources
  turningMachine1 : $bdroot/turningMachine  turning_time=turning_time  ap_ug=0.5  ap_og=1.5  P_ap=0.6  f_ug=0.1  f_og=0.5  P_f=0.4  vc_ug=150  vc_og=350  P_vc=0.5  ap=ap  f=f  vc=vc  tauInt=tauInt  tauCont=tauCont  tau=[0,1]  debug=debug
  turningMachine2 : $bdroot/turningMachine  turning_time=turning_time  ap_ug=0.5  ap_og=1.5  P_ap=0.6  f_ug=0.1  f_og=0.5  P_f=0.4  vc_ug=150  vc_og=350  P_vc=0.5  ap=ap  f=f  vc=vc  tauInt=tauInt  tauCont=tauCont  tau=[0,1]  debug=debug
  turningMachine3 : $bdroot/turningMachine  turning_time=turning_time  ap_ug=0.5  ap_og=1.5  P_ap=0.6  f_ug=0.1  f_og=0.5  P_f=0.4  vc_ug=150  vc_og=350  P_vc=0.5  ap=ap  f=f  vc=vc  tauInt=tauInt  tauCont=tauCont  tau=[0,1]  debug=debug
  out : Outport
  release : Outport  Port=2
  working : Outport  Port=3
  nq : Outport  Port=4
  e : Outport  Port=5
  p : Outport  Port=6
  util : Outport  Port=7
  wires:
  turningMachine2/2 -> combineData/2, input_queue/4
  turningMachine1/2 -> combineData/1, input_queue/3
  turningMachine1/1 -> combine3/1
  turningMachine2/1 -> combine3/2
  turningMachine3/1 -> combine3/3
  combine3/1 -> out/1
  turningMachine3/2 -> combineData/3, input_queue/5
  enable/1 -> input_queue/1
  in/1 -> input_queue/2
  input_queue/1 -> am_comparator/1, nq/1
  input_queue/2 -> turningMachine1/1
  input_queue/3 -> turningMachine2/1
  input_queue/4 -> turningMachine3/1
  turningMachine1/3 -> combineData/4
  turningMachine1/4 -> combineData/7
  turningMachine2/3 -> combineData/5
  turningMachine2/4 -> combineData/8
  turningMachine3/3 -> combineData/6
  turningMachine3/4 -> combineData/9
  combineData/1 -> working/1
  combineData/3 -> p/1
  combineData/2 -> e/1
  combineData/4 -> util/1
  am_comparator/1 -> release/1
  max_fifo/1 -> am_comparator/2

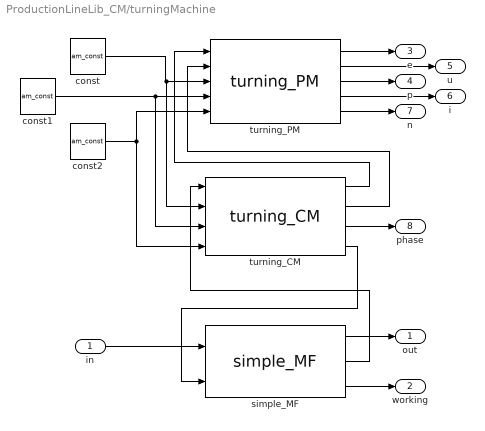
== system ProductionLineLib_CM/turningMachine ==
  in : Inport
  const : NSA_DEVS_SOURCES/am_const  value=ap  sendTime=[0,1]  debug=0
      settings: SourceProductName=Sources
  const1 : NSA_DEVS_SOURCES/am_const  value=f  sendTime=[0,1]  debug=0
      settings: SourceProductName=Sources
  const2 : NSA_DEVS_SOURCES/am_const  value=vc  sendTime=[0,1]  debug=0
      settings: SourceProductName=Sources
  simple_MF : $bdroot/simple_MF  tau=tau  debug=debug
  turning_CM : $bdroot/turning_CM  turning_time=turning_time  ap_ug=ap_ug  f_ug=f_ug  vc_ug=vc_ug  ap_og=ap_og  f_og=f_og  vc_og=vc_og  tau=tauCont  debug=debug
  turning_PM : $bdroot/turning_PM  R=6  L=0.2  J=0.052  b=0.015  K=0.15  vcc=150  vcc_load=30  load=0.75/200  ap_ug=ap_ug  f_ug=f_ug  vc_ug=vc_ug  ap_og=ap_og  f_og=f_og  vc_og=vc_og  P_ap=P_ap  P_f=P_f  P_vc=P_vc  tauInt=tauInt  tau=tau  debug=debug
  out : Outport
  working : Outport  Port=2
  e : Outport  Port=3
  p : Outport  Port=4
  u : Outport  Port=5
  i : Outport  Port=6
  n : Outport  Port=7
  phase : Outport  Port=8
  wires:
  simple_MF/2 -> turning_CM/1
  turning_CM/4 -> simple_MF/2
  turning_CM/2 -> turning_PM/2
  turning_CM/1 -> turning_PM/1
  turning_PM/3 -> p/1
  turning_PM/1 -> e/1
  simple_MF/3 -> working/1
  simple_MF/1 -> out/1
  in/1 -> simple_MF/1
  turning_PM/2 -> u/1
  turning_PM/4 -> i/1
  turning_PM/5 -> n/1
  turning_CM/3 -> phase/1
  const1/1 -> turning_CM/3, turning_PM/4
  const2/1 -> turning_PM/5, turning_CM/4
  const/1 -> turning_CM/2, turning_PM/3

== system ProductionLineLib_CM/turningMotorI ==
  u : Inport
  n : Inport  Port=2
  add3 : NSA_DEVS_MATH_OPERATIONS/am_add3  tau=tau  debug=debug
      settings: SourceProductName=Math Operations
  gain : NSA_DEVS_MATH_OPERATIONS/am_gain  g=1/L  tau=[0,1]  debug=debug
      settings: SourceProductName=Math Operations
  gain1 : NSA_DEVS_MATH_OPERATIONS/am_gain  g=-K  tau=tau  debug=debug
      settings: SourceProductName=Math Operations
  gain2 : NSA_DEVS_MATH_OPERATIONS/am_gain  g=-R  tau=[0,1]  debug=debug
      settings: SourceProductName=Math Operations
  hIntegrator : NSA_DEVS_QSS/am_hIntegrator  dq=5  epsilon=100  X0=0  tau=tauInt  debug=debug
      settings: SourceProductName=QSS
  i : Outport
  wires:
  n/1 -> gain1/1
  add3/1 -> gain/1
  gain/1 -> hIntegrator/1
  gain1/1 -> add3/3
  hIntegrator/1 -> i/1, gain2/1
  u/1 -> add3/2
  gain2/1 -> add3/1

== system ProductionLineLib_CM/turningMotorN ==
  i : Inport
  turning : Inport  Port=2
  add3 : NSA_DEVS_MATH_OPERATIONS/am_add3  tau=[0,1]  debug=debug
      settings: SourceProductName=Math Operations
  const : NSA_DEVS_SOURCES/am_const  value=load  sendTime=[0,1]  debug=debug
      settings: SourceProductName=Sources
  gain : NSA_DEVS_MATH_OPERATIONS/am_gain  g=-1  tau=[0,1]  debug=debug
      settings: SourceProductName=Math Operations
  gain1 : NSA_DEVS_MATH_OPERATIONS/am_gain  g=K  tau=tau  debug=debug
      settings: SourceProductName=Math Operations
  gain2 : NSA_DEVS_MATH_OPERATIONS/am_gain  g=1/J  tau=[0,1]  debug=debug
      settings: SourceProductName=Math Operations
  gain3 : NSA_DEVS_MATH_OPERATIONS/am_gain  g=30/pi  tau=[0,1]  debug=debug
      settings: SourceProductName=Math Operations
  gain4 : NSA_DEVS_MATH_OPERATIONS/am_gain  g=-b  tau=[0,1]  debug=debug
      settings: SourceProductName=Math Operations
  hIntegrator : NSA_DEVS_QSS/am_hIntegrator  dq=50  epsilon=100  X0=0  tau=tauInt  debug=debug
      settings: SourceProductName=QSS
  mult3 : NSA_DEVS_MATH_OPERATIONS/am_mult3  tau=tau  debug=debug
      settings: SourceProductName=Math Operations
  n : Outport
  n_rad : Outport  Port=2
  wires:
  add3/1 -> gain2/1
  turning/1 -> mult3/2
  const/1 -> mult3/1
  mult3/1 -> gain/1
  gain4/1 -> add3/3
  hIntegrator/1 -> gain3/1, n_rad/1, mult3/3, gain4/1
  gain3/1 -> n/1
  gain2/1 -> hIntegrator/1
  gain/1 -> add3/2
  i/1 -> gain1/1
  gain1/1 -> add3/1

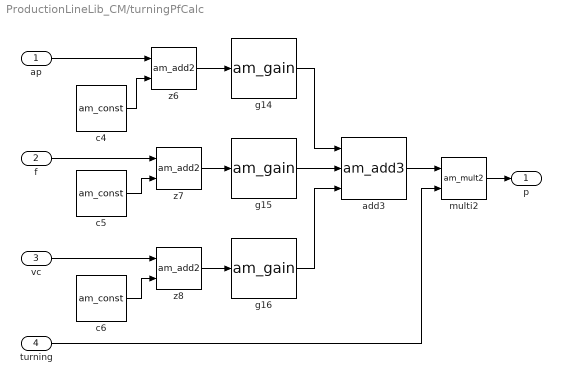
== system ProductionLineLib_CM/turningPfCalc ==
  ap : Inport
  f : Inport  Port=2
  vc : Inport  Port=3
  turning : Inport  Port=4
  add3 : NSA_DEVS_MATH_OPERATIONS/am_add3  tau=[0,1]  debug=debug
      settings: SourceProductName=Math Operations
  c4 : NSA_DEVS_SOURCES/am_const  value=-ap_ug  sendTime=[0,1]  debug=debug
      settings: SourceProductName=Sources
  c5 : NSA_DEVS_SOURCES/am_const  value=-f_ug  sendTime=[0,1]  debug=debug
      settings: SourceProductName=Sources
  c6 : NSA_DEVS_SOURCES/am_const  value=-vc_ug  sendTime=[0,1]  debug=debug
      settings: SourceProductName=Sources
  g14 : NSA_DEVS_MATH_OPERATIONS/am_gain  g=1/(ap_og - ap_ug)*P_ap  tau=[0,1]  debug=debug
      settings: SourceProductName=Math Operations
  g15 : NSA_DEVS_MATH_OPERATIONS/am_gain  g=1/(f_og - f_ug)*P_f  tau=[0,1]  debug=debug
      settings: SourceProductName=Math Operations
  g16 : NSA_DEVS_MATH_OPERATIONS/am_gain  g=1/(vc_og - vc_ug)*P_vc  tau=[0,1]  debug=debug
      settings: SourceProductName=Math Operations
  multi2 : NSA_DEVS_MATH_OPERATIONS/am_mult2  tau=tau  debug=debug
      settings: SourceProductName=Math Operations
  z6 : NSA_DEVS_MATH_OPERATIONS/am_add2  tau=tau  debug=debug
      settings: SourceProductName=Math Operations
  z7 : NSA_DEVS_MATH_OPERATIONS/am_add2  tau=tau  debug=debug
      settings: SourceProductName=Math Operations
  z8 : NSA_DEVS_MATH_OPERATIONS/am_add2  tau=tau  debug=debug
      settings: SourceProductName=Math Operations
  p : Outport
  wires:
  g14/1 -> add3/1
  g15/1 -> add3/2
  c6/1 -> z8/2
  z8/1 -> g16/1
  g16/1 -> add3/3
  turning/1 -> multi2/2
  z6/1 -> g14/1
  c4/1 -> z6/2
  z7/1 -> g15/1
  multi2/1 -> p/1
  c5/1 -> z7/2
  vc/1 -> z8/1
  add3/1 -> multi2/1
  ap/1 -> z6/1
  f/1 -> z7/1

== system ProductionLineLib_CM/turningPowerCalc ==
  p_in : Inport
  u_in : Inport  Port=2
  i_in : Inport  Port=3
  add2 : NSA_DEVS_MATH_OPERATIONS/am_add2  tau=tau  debug=debug
      settings: SourceProductName=Math Operations
  gain : NSA_DEVS_MATH_OPERATIONS/am_gain  g=1/1000  tau=[0,1]  debug=debug
      settings: SourceProductName=Math Operations
  gain1 : NSA_DEVS_MATH_OPERATIONS/am_gain  g=1/3600  tau=[0,1]  debug=debug
      settings: SourceProductName=Math Operations
  hIntegrator : NSA_DEVS_QSS/am_hIntegrator  dq=0.1  epsilon=0.2  X0=0  tau=tauInt  debug=debug
      settings: SourceProductName=QSS
  multi2 : NSA_DEVS_MATH_OPERATIONS/am_mult2  tau=tau  debug=debug
      settings: SourceProductName=Math Operations
  saturation : NSA_DEVS_MATH_OPERATIONS/am_saturation  ll=0  ul=Inf  tau=tau  debug=debug
      settings: SourceProductName=Math Operations
  i_out : Outport
  p_out : Outport  Port=2
  e_out : Outport  Port=3
  wires:
  multi2/1 -> gain/1
  saturation/1 -> i_out/1, multi2/1
  u_in/1 -> multi2/2
  i_in/1 -> saturation/1
  p_in/1 -> add2/1
  gain/1 -> add2/2
  add2/1 -> p_out/1, gain1/1
  hIntegrator/1 -> e_out/1
  gain1/1 -> hIntegrator/1
